simulink model "MdXXHolderChk"  (R2024b)
settings: Solver=FixedStepDiscrete  StartTime=0.0  StopTime=10.0  FixedStep=0.01  RelTol=1e-3
undefined symbols (not defined in the file or in its folder): KeSMSwAcsMd32SecRwLtStBkReclnUpwdDnwdPos1_Val, KeSMSwAcsMd53SecRwRtStBkReclnUpwdDnwdPos1_Val, SeatChldLkSt
libraries: simulink x41
(part 2 of 5)

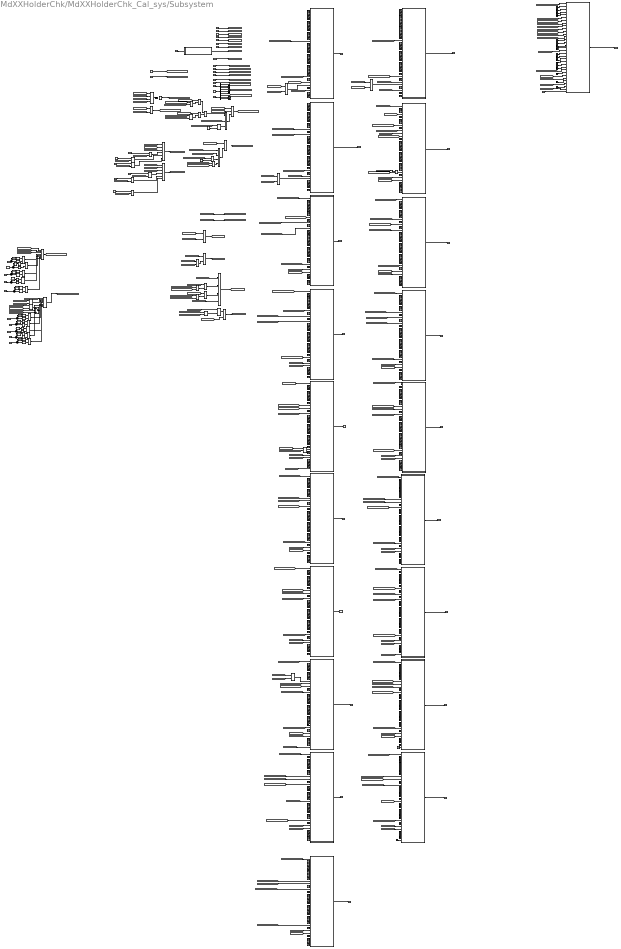
== system MdXXHolderChk/MdXXHolderChk_Cal_sys/Subsystem ==
  note: 零重力模式，二排任意一个电机没到位，模式直接停止
  ChldLkRspFlgL_Val_read : Inport
  ChldLkRspFlgR_Val_read : Inport  Port=2
  PassSeatOccupied_Val_read : Inport  Port=3
  R3LMdSeatOccupied_Val_read : Inport  Port=4
  R3RMdSeatOccupied_Val_read : Inport  Port=5
  R2LMdSeatOccupied_Val_read : Inport  Port=6
  R2RMdSeatOccupied_Val_read : Inport  Port=7
  StNumFlg_Is7s_read : Inport  Port=8
  IfVeSMSbThdRwLtStCshnFldUpwdDnwdMovConfig_Val_read : Inport  Port=9
  IfVeSMSuThdRwLtStCshnFldUpwdDnwdPos_Val_read : Inport  Port=10
  IfVeSMSuThdRwRtStCshnFldUpwdDnwdPos_Val_read : Inport  Port=11
  IfVeSMSbThdRwRtStCshnFldUpwdDnwdMovConfig_Val_read : Inport  Port=12
  IfVeSMSuSecRwLtStBkReclnUpwdDnwdPos_Val_read : Inport  Port=13
  IfVeSMSuSecRwRtStBkReclnUpwdDnwdPos_Val_read : Inport  Port=14
  Md8R2LBkReclnUpwdDnwdTrgtPosCalib_TrgtPosArray_read : Inport  Port=15
  Md8R2RBkReclnUpwdDnwdTrgtPosCalib_TrgtPosArray_read : Inport  Port=16
  Md9R2RBkReclnUpwdDnwdTrgtPosCalib_TrgtPosArray_read : Inport  Port=17
  ThdRwLtStChldLkReq_Val_read : Inport  Port=18
  KeSMSwAcsMd32SecRwLtStBkReclnUpwdDnwdPos1 : Inport  Port=19
  KeSMSwAcsMd53SecRwRtStBkReclnUpwdDnwdPos1 : Inport  Port=20
  Md61PassStTrgtIsFld_Val_read : Inport  Port=21
  Md61ThdRwLtStTrgtIsFld_Val_read : Inport  Port=22
  Md61ThdRwRtStTrgtIsFld_Val_read : Inport  Port=23
  Md62PassStTrgtIsFld_Val_read : Inport  Port=24
  Md62ThdRwLtStTrgtIsFld_Val_read : Inport  Port=25
  Md62ThdRwRtStTrgtIsFld_Val_read : Inport  Port=26
  BkReclinctrlquitflagL_Val_read : Inport  Port=27
  BkReclnquitflag_Val_read : Inport  Port=28
  FwdBkwdquitflag_Val_read : Inport  Port=29
  FwdBkwdquitflagL_Val_read : Inport  Port=30
  LgrstDwwdUpwdquitflagL_Val_read : Inport  Port=31
  LgrstInwdOtwdquitflagL_Val_read : Inport  Port=32
  LgrstInwrdOutwdquitflag_Val_read : Inport  Port=33
  LgrstUpwdDnwdquitflag_Val_read : Inport  Port=34
  Zeroquitflag_Val_read : Inport  Port=35
  zeroquitflagL_Val_read : Inport  Port=36
  modestate32_Val_read : Inport  Port=37
  Compare To Constant{,2,4,6,8,10,12,14,16,18} (10 alike) : simulink/Logic and Bit Operations/Compare To Constant  relop===  const=0  OutDataTypeStr=boolean
  Compare To Constant{1,3,5,7,9,11,13,15,17,19} (10 alike) : simulink/Logic and Bit Operations/Compare To Constant  relop===  const=1  OutDataTypeStr=boolean
  Constant : Constant  Value=0  OutDataTypeStr=boolean
  Constant1 : Constant  Value=40  OutDataTypeStr=uint16
  Constant3 : Constant  Value=40  OutDataTypeStr=uint16
  Demux : Demux  Outputs=3
  Demux1 : Demux  Outputs=3
  Demux2 : Demux  Outputs=3
  Ground{,1..3,8..11,13..18,20..21,23} (17 alike) : Ground
  Ground_{1..26,28..41,43,45..56,58,61..64,66..72,75,77..88,90,93..96,98..104,107,109..113,115..120,122,125..127,130..135,139,141..152,154,157..159,162..168,171,173..184,186,189..192,194..200,203,205..216,218,221..224,226..231,233,235,237..248,250,253..256,258..263,265,267,269..280,282,285..288,291,293..295,297,301..312,314,317..331,333..344,346,349,351..352,354..359,361,363,365..376,378,381..384,386..391,393,395,397..408,410,413..416,418..424,427,429..440,442,445..447,450..456,459,461..472,474,477..480,482..488,491,493..504,506,509..512,514..519,523,525..535,538,541..543,546..552,555,557..561,563..568,570,573..576,578..583,585,587,589..600,602,605..607} (472 alike) : Ground
  Logical Operator{,1,5,8,10..11,13,16..17,46,79,82,86} (13 alike) : Logic  Operator=OR  AllPortsSameDT=off  OutDataTypeStr=boolean
  Logical Operator{6..7,12,14..15,18,20..34,45,83} (23 alike) : Logic  AllPortsSameDT=off  OutDataTypeStr=boolean
  Logical Operator19 : Logic  Operator=OR  Inputs=6  AllPortsSameDT=off  OutDataTypeStr=boolean
  Logical Operator2 : Logic  Operator=OR  Inputs=8  AllPortsSameDT=off  OutDataTypeStr=boolean
  Logical Operator3 : Logic  Operator=OR  Inputs=4  AllPortsSameDT=off  OutDataTypeStr=boolean
  Logical Operator4 : Logic  Operator=OR  Inputs=6  AllPortsSameDT=off  OutDataTypeStr=boolean
  Logical Operator78 : Logic  Inputs=4  AllPortsSameDT=off  OutDataTypeStr=boolean
  Logical Operator81 : Logic  Operator=OR  Inputs=8  AllPortsSameDT=off  OutDataTypeStr=boolean
  Logical Operator84 : Logic  Operator=OR  Inputs=3  AllPortsSameDT=off  OutDataTypeStr=boolean
  Logical Operator85 : Logic  Inputs=3  AllPortsSameDT=off  OutDataTypeStr=boolean
  Logical Operator9 : Logic  Operator=OR  Inputs=4  AllPortsSameDT=off  OutDataTypeStr=boolean
  Relational Operator{1..8} (8 alike) : RelationalOperator  Operator=>  OutDataTypeStr=boolean  RndMeth=Simplest  InputSameDT=off
  Subsystem : Subsystem
  Subsystem1 : Subsystem
  Subsystem10 : Subsystem
  Subsystem11 : Subsystem
  Subsystem12 : Subsystem
  Subsystem13 : Subsystem
  Subsystem14 : Subsystem
  Subsystem15 : Subsystem
  Subsystem16 : Subsystem
  Subsystem17 : Subsystem
  Subsystem18 : Subsystem
  Subsystem19 : Subsystem
  Subsystem2 : Subsystem
  Subsystem20 : Subsystem
  Subsystem3 : Subsystem
  Subsystem4 : Subsystem
  Subsystem5 : Subsystem
  Subsystem6 : Subsystem
  Subsystem7 : Subsystem
  Subsystem8 : Subsystem
  Subsystem9 : Subsystem
  Switch19 : Switch  Criteria=u2 > Threshold  SaturateOnIntegerOverflow=off  InputSameDT=off
  Terminator{,1..6} (7 alike) : Terminator
  Unit Delay{,1..9} (10 alike) : UnitDelay  SampleTime=-1  HasFrameUpgradeWarning=on
  MdXXPassStBkReclnHolderInfo_Val_write : Outport  VectorParamsAs1DForOutWhenUnconnected=off
      settings: EnsureOutportIsVirtual=on
  MdXXPassStCshnFldHolderInfo_Val_write : Outport  Port=2  VectorParamsAs1DForOutWhenUnconnected=off
      settings: EnsureOutportIsVirtual=on
  MdXXPassStFwdBkwdHolderInfo_Val_write : Outport  Port=3  VectorParamsAs1DForOutWhenUnconnected=off
      settings: EnsureOutportIsVirtual=on
  MdXXSecRwLtStBkReclnHolderInfo_Val_write : Outport  Port=4  VectorParamsAs1DForOutWhenUnconnected=off
      settings: EnsureOutportIsVirtual=on
  MdXXSecRwLtStFwdBkwdHolderInfo_Val_write : Outport  Port=5  VectorParamsAs1DForOutWhenUnconnected=off
      settings: EnsureOutportIsVirtual=on
  MdXXSecRwLtStLgrstInwdOtwdHolderInfo_Val_write : Outport  Port=6  VectorParamsAs1DForOutWhenUnconnected=off
      settings: EnsureOutportIsVirtual=on
  MdXXSecRwLtStLgrstUpwdDnwdHolderInfo_Val_write : Outport  Port=7  VectorParamsAs1DForOutWhenUnconnected=off
      settings: EnsureOutportIsVirtual=on
  MdXXSecRwLtStZeroHolderInfo_Val_write : Outport  Port=8  VectorParamsAs1DForOutWhenUnconnected=off
      settings: EnsureOutportIsVirtual=on
  MdXXSecRwRtStBkReclnEnHolderInfo_Val_write : Outport  Port=9  VectorParamsAs1DForOutWhenUnconnected=off
      settings: EnsureOutportIsVirtual=on
  MdXXSecRwRtStFwdBkwdHolderInfo_Val_write : Outport  Port=10  VectorParamsAs1DForOutWhenUnconnected=off
      settings: EnsureOutportIsVirtual=on
  MdXXSecRwRtStLgrstInwdOtwdHolderInfo_Val_write : Outport  Port=11  VectorParamsAs1DForOutWhenUnconnected=off
      settings: EnsureOutportIsVirtual=on
  MdXXSecRwRtStLgrstUpwdDnwdHolderInfo_Val_write : Outport  Port=12  VectorParamsAs1DForOutWhenUnconnected=off
      settings: EnsureOutportIsVirtual=on
  MdXXSecRwRtStZeroHolderInfo_Val_write : Outport  Port=13  VectorParamsAs1DForOutWhenUnconnected=off
      settings: EnsureOutportIsVirtual=on
  MdXXThdRwLtStBkReclnHolderInfo_Val_write : Outport  Port=14  VectorParamsAs1DForOutWhenUnconnected=off
      settings: EnsureOutportIsVirtual=on
  MdXXThdRwLtStCshnFldHolderInfo_Val_write : Outport  Port=15  VectorParamsAs1DForOutWhenUnconnected=off
      settings: EnsureOutportIsVirtual=on
  MdXXThdRwLtStFwdBkwdHolderInfo_Val_write : Outport  Port=16  VectorParamsAs1DForOutWhenUnconnected=off
      settings: EnsureOutportIsVirtual=on
  MdXXThdRwRtStBkReclnHolderInfo_Val_write : Outport  Port=17  VectorParamsAs1DForOutWhenUnconnected=off
      settings: EnsureOutportIsVirtual=on
  MdXXThdRwRtStCshnFldHolderInfo_Val_write : Outport  Port=18  VectorParamsAs1DForOutWhenUnconnected=off
      settings: EnsureOutportIsVirtual=on
  MdXXThdRwRtStFwdBkwdHolderInfo_Val_write : Outport  Port=19  VectorParamsAs1DForOutWhenUnconnected=off
      settings: EnsureOutportIsVirtual=on
  MdXXHolderInfo_Val_write : Outport  Port=20  VectorParamsAs1DForOutWhenUnconnected=off
      settings: EnsureOutportIsVirtual=on
  wires:
  Subsystem/1(MdXXHolder) -> MdXXPassStBkReclnHolderInfo_Val_write/1
  Subsystem18/1(MdXXHolder) -> MdXXPassStCshnFldHolderInfo_Val_write/1
  Subsystem1/1(MdXXHolder) -> MdXXPassStFwdBkwdHolderInfo_Val_write/1
  Subsystem17/1(MdXXHolder) -> MdXXSecRwLtStBkReclnHolderInfo_Val_write/1
  Subsystem2/1(MdXXHolder) -> MdXXSecRwLtStFwdBkwdHolderInfo_Val_write/1
  Subsystem16/1(MdXXHolder) -> MdXXSecRwLtStLgrstInwdOtwdHolderInfo_Val_write/1
  Subsystem3/1(MdXXHolder) -> MdXXSecRwLtStLgrstUpwdDnwdHolderInfo_Val_write/1
  Subsystem15/1(MdXXHolder) -> MdXXSecRwLtStZeroHolderInfo_Val_write/1
  Subsystem4/1(MdXXHolder) -> MdXXSecRwRtStBkReclnEnHolderInfo_Val_write/1
  Subsystem14/1(MdXXHolder) -> MdXXSecRwRtStFwdBkwdHolderInfo_Val_write/1
  Subsystem5/1(MdXXHolder) -> MdXXSecRwRtStLgrstInwdOtwdHolderInfo_Val_write/1
  Subsystem13/1(MdXXHolder) -> MdXXSecRwRtStLgrstUpwdDnwdHolderInfo_Val_write/1
  Subsystem6/1(MdXXHolder) -> MdXXSecRwRtStZeroHolderInfo_Val_write/1
  Subsystem9/1(MdXXHolder) -> MdXXThdRwLtStBkReclnHolderInfo_Val_write/1
  Subsystem7/1(MdXXHolder) -> MdXXThdRwLtStCshnFldHolderInfo_Val_write/1
  Subsystem12/1(MdXXHolder) -> MdXXThdRwLtStFwdBkwdHolderInfo_Val_write/1
  Subsystem8/1(MdXXHolder) -> MdXXThdRwRtStBkReclnHolderInfo_Val_write/1
  Subsystem11/1(MdXXHolder) -> MdXXThdRwRtStCshnFldHolderInfo_Val_write/1
  Subsystem10/1(MdXXHolder) -> MdXXThdRwRtStFwdBkwdHolderInfo_Val_write/1
  ChldLkRspFlgL_Val_read/1 -> [ChldLkRspFlgL]
  ChldLkRspFlgR_Val_read/1 -> [ChldLkRspFlgR]
  PassSeatOccupied_Val_read/1 -> [PassSeatOccupied]
  R3LMdSeatOccupied_Val_read/1 -> [R3LMdSeatOccupied]
  R3RMdSeatOccupied_Val_read/1 -> [R3RMdSeatOccupied]
  Ground_1/1 -> Subsystem/1(Md1HoldReq)
  Ground_2/1 -> Subsystem/2(Md2HoldReq)
  Ground_3/1 -> Subsystem/3(Md3HoldReq)
  Ground_4/1 -> Subsystem/4(Md4HoldReq)
  Ground_5/1 -> Subsystem/5(Md5HoldReq)
  Ground_6/1 -> Subsystem/6(Md6HoldReq)
  Ground_7/1 -> Subsystem/7(Md7HoldReq)
  Ground_8/1 -> Subsystem/8(Md8HoldReq)
  Ground_9/1 -> Subsystem/9(Md9HoldReq)
  Ground_10/1 -> Subsystem/10(Md10HoldReq)
  Ground_11/1 -> Subsystem/11(Md11HoldReq)
  Ground_13/1 -> Subsystem/13(Md13HoldReq)
  Ground_14/1 -> Subsystem/14(Md14HoldReq)
  Ground_15/1 -> Subsystem/15(Md15HoldReq)
  Ground_16/1 -> Subsystem/16(Md16HoldReq)
  Ground_17/1 -> Subsystem/17(Md17HoldReq)
  Ground_18/1 -> Subsystem/18(Md18HoldReq)
  Ground_19/1 -> Subsystem/19(Md19HoldReq)
  Ground_20/1 -> Subsystem/20(Md20HoldReq)
  Ground_21/1 -> Subsystem/21(Md21HoldReq)
  Ground_22/1 -> Subsystem/22(Md22HoldReq)
  Ground_23/1 -> Subsystem/23(Md23HoldReq)
  Ground_24/1 -> Subsystem/24(Md24HoldReq)
  [Md56Stop] -> Subsystem/25(Md25HoldReq)
  Ground_26/1 -> Subsystem/26(Md26HoldReq)
  Ground_29/1 -> Subsystem/29(Md29HoldReq)
  [PassSeatOccupied] -> Subsystem/30(Md30HoldReq)
  Ground_31/1 -> Subsystem/31(Md31HoldReq)
  Ground_32/1 -> Subsystem/32(Md32HoldReq)
  Ground_33/1 -> Subsystem1/1(Md1HoldReq)
  Ground_34/1 -> Subsystem1/2(Md2HoldReq)
  Ground_35/1 -> Subsystem1/3(Md3HoldReq)
  Ground_36/1 -> Subsystem1/4(Md4HoldReq)
  Ground_37/1 -> Subsystem1/5(Md5HoldReq)
  Ground_38/1 -> Subsystem1/6(Md6HoldReq)
  Ground_39/1 -> Subsystem1/7(Md7HoldReq)
  Ground_40/1 -> Subsystem1/8(Md8HoldReq)
  Ground_41/1 -> Subsystem1/9(Md9HoldReq)
  Ground_43/1 -> Subsystem1/11(Md11HoldReq)
  Ground_45/1 -> Subsystem1/13(Md13HoldReq)
  Ground_46/1 -> Subsystem1/14(Md14HoldReq)
  Ground_47/1 -> Subsystem1/15(Md15HoldReq)
  Ground_48/1 -> Subsystem1/16(Md16HoldReq)
  Ground_49/1 -> Subsystem1/17(Md17HoldReq)
  Ground_50/1 -> Subsystem1/18(Md18HoldReq)
  Ground_51/1 -> Subsystem1/19(Md19HoldReq)
  Ground_52/1 -> Subsystem1/20(Md20HoldReq)
  Ground_53/1 -> Subsystem1/21(Md21HoldReq)
  Ground_54/1 -> Subsystem1/22(Md22HoldReq)
  Ground_55/1 -> Subsystem1/23(Md23HoldReq)
  Ground_56/1 -> Subsystem1/24(Md24HoldReq)
  [Md56Stop] -> Subsystem1/25(Md25HoldReq)
  Ground_58/1 -> Subsystem1/26(Md26HoldReq)
  [Md27Stop] -> Subsystem1/27(Md27HoldReq)
  Ground_61/1 -> Subsystem1/29(Md29HoldReq)
  Ground_62/1 -> Subsystem1/30(Md30HoldReq)
  Ground_63/1 -> Subsystem1/31(Md31HoldReq)
  Ground_64/1 -> Subsystem1/32(Md32HoldReq)
  [Md1Stop] -> Subsystem10/1(Md1HoldReq)
  Ground_66/1 -> Subsystem10/2(Md2HoldReq)
  Ground_67/1 -> Subsystem10/3(Md3HoldReq)
  Ground_68/1 -> Subsystem10/4(Md4HoldReq)
  Ground_69/1 -> Subsystem10/5(Md5HoldReq)
  Ground_70/1 -> Subsystem10/6(Md6HoldReq)
  Ground_71/1 -> Subsystem10/7(Md7HoldReq)
  Ground_72/1 -> Subsystem10/8(Md8HoldReq)
  [Md10Stop] -> Subsystem10/10(Md10HoldReq)
  Ground_75/1 -> Subsystem10/11(Md11HoldReq)
  Ground_77/1 -> Subsystem10/13(Md13HoldReq)
  Ground_78/1 -> Subsystem10/14(Md14HoldReq)
  Ground_79/1 -> Subsystem10/15(Md15HoldReq)
  Ground_80/1 -> Subsystem10/16(Md16HoldReq)
  Ground_81/1 -> Subsystem10/17(Md17HoldReq)
  Ground_82/1 -> Subsystem10/18(Md18HoldReq)
  Ground_83/1 -> Subsystem10/19(Md19HoldReq)
  Ground_84/1 -> Subsystem10/20(Md20HoldReq)
  Ground_85/1 -> Subsystem10/21(Md21HoldReq)
  Ground_86/1 -> Subsystem10/22(Md22HoldReq)
  Ground_87/1 -> Subsystem10/23(Md23HoldReq)
  Ground_88/1 -> Subsystem10/24(Md24HoldReq)
  [Md56Stop] -> Subsystem10/25(Md25HoldReq)
  Ground_90/1 -> Subsystem10/26(Md26HoldReq)
  Ground_93/1 -> Subsystem10/29(Md29HoldReq)
  Ground_94/1 -> Subsystem10/30(Md30HoldReq)
  Ground_95/1 -> Subsystem10/31(Md31HoldReq)
  Ground_96/1 -> Subsystem10/32(Md32HoldReq)
  [Md1Stop] -> Subsystem11/1(Md1HoldReq)
  Ground_98/1 -> Subsystem11/2(Md2HoldReq)
  Ground_99/1 -> Subsystem11/3(Md3HoldReq)
  Ground_100/1 -> Subsystem11/4(Md4HoldReq)
  Ground_101/1 -> Subsystem11/5(Md5HoldReq)
  Ground_102/1 -> Subsystem11/6(Md6HoldReq)
  Ground_103/1 -> Subsystem11/7(Md7HoldReq)
  Ground_104/1 -> Subsystem11/8(Md8HoldReq)
  [Md10Stop] -> Subsystem11/10(Md10HoldReq)
  Ground_107/1 -> Subsystem11/11(Md11HoldReq)
  Ground_109/1 -> Subsystem11/13(Md13HoldReq)
  Ground_110/1 -> Subsystem11/14(Md14HoldReq)
  Ground_111/1 -> Subsystem11/15(Md15HoldReq)
  Ground_112/1 -> Subsystem11/16(Md16HoldReq)
  Ground_113/1 -> Subsystem11/17(Md17HoldReq)
  [R3RMdSeatOccupied] -> Subsystem11/18(Md18HoldReq)
  Ground_115/1 -> Subsystem11/19(Md19HoldReq)
  Ground_116/1 -> Subsystem11/20(Md20HoldReq)
  Ground_117/1 -> Subsystem11/21(Md21HoldReq)
  Ground_118/1 -> Subsystem11/22(Md22HoldReq)
  Ground_119/1 -> Subsystem11/23(Md23HoldReq)
  Ground_120/1 -> Subsystem11/24(Md24HoldReq)
  [Md56Stop] -> Subsystem11/25(Md25HoldReq)
  Ground_122/1 -> Subsystem11/26(Md26HoldReq)
  Ground_125/1 -> Subsystem11/29(Md29HoldReq)
  Ground_126/1 -> Subsystem11/30(Md30HoldReq)
  Ground_127/1 -> Subsystem11/31(Md31HoldReq)
  [Md1Stop] -> Subsystem12/1(Md1HoldReq)
  Ground_130/1 -> Subsystem12/2(Md2HoldReq)
  Ground_131/1 -> Subsystem12/3(Md3HoldReq)
  Ground_132/1 -> Subsystem12/4(Md4HoldReq)
  Ground_133/1 -> Subsystem12/5(Md5HoldReq)
  Ground_134/1 -> Subsystem12/6(Md6HoldReq)
  Ground_135/1 -> Subsystem12/7(Md7HoldReq)
  [Md9Stop] -> Subsystem12/9(Md9HoldReq)
  [Md10Stop] -> Subsystem12/10(Md10HoldReq)
  Ground_139/1 -> Subsystem12/11(Md11HoldReq)
  Ground_141/1 -> Subsystem12/13(Md13HoldReq)
  Ground_142/1 -> Subsystem12/14(Md14HoldReq)
  Ground_143/1 -> Subsystem12/15(Md15HoldReq)
  Ground_144/1 -> Subsystem12/16(Md16HoldReq)
  Ground_145/1 -> Subsystem12/17(Md17HoldReq)
  Ground_146/1 -> Subsystem12/18(Md18HoldReq)
  Ground_147/1 -> Subsystem12/19(Md19HoldReq)
  Ground_148/1 -> Subsystem12/20(Md20HoldReq)
  Ground_149/1 -> Subsystem12/21(Md21HoldReq)
  Ground_150/1 -> Subsystem12/22(Md22HoldReq)
  Ground_151/1 -> Subsystem12/23(Md23HoldReq)
  Ground_152/1 -> Subsystem12/24(Md24HoldReq)
  [Md56Stop] -> Subsystem12/25(Md25HoldReq)
  Ground_154/1 -> Subsystem12/26(Md26HoldReq)
  Ground_157/1 -> Subsystem12/29(Md29HoldReq)
  Ground_158/1 -> Subsystem12/30(Md30HoldReq)
  Ground_159/1 -> Subsystem12/31(Md31HoldReq)
  Ground_28/1 -> Subsystem12/32(Md32HoldReq)
  [Md1Stop] -> Subsystem13/1(Md1HoldReq)
  Ground_162/1 -> Subsystem13/2(Md2HoldReq)
  Ground_163/1 -> Subsystem13/3(Md3HoldReq)
  Ground_164/1 -> Subsystem13/4(Md4HoldReq)
  Ground_165/1 -> Subsystem13/5(Md5HoldReq)
  Ground_166/1 -> Subsystem13/6(Md6HoldReq)
  Ground_167/1 -> Subsystem13/7(Md7HoldReq)
  Ground_168/1 -> Subsystem13/8(Md8HoldReq)
  [Md9Stop] -> Subsystem13/9(Md9HoldReq)
  [Md10Stop] -> Subsystem13/10(Md10HoldReq)
  Ground_171/1 -> Subsystem13/11(Md11HoldReq)
  Ground_173/1 -> Subsystem13/13(Md13HoldReq)
  Ground_174/1 -> Subsystem13/14(Md14HoldReq)
  Ground_175/1 -> Subsystem13/15(Md15HoldReq)
  Ground_176/1 -> Subsystem13/16(Md16HoldReq)
  Ground_177/1 -> Subsystem13/17(Md17HoldReq)
  Ground_178/1 -> Subsystem13/18(Md18HoldReq)
  Ground_179/1 -> Subsystem13/19(Md19HoldReq)
  Ground_180/1 -> Subsystem13/20(Md20HoldReq)
  Ground_181/1 -> Subsystem13/21(Md21HoldReq)
  Ground_182/1 -> Subsystem13/22(Md22HoldReq)
  Ground_183/1 -> Subsystem13/23(Md23HoldReq)
  Ground_184/1 -> Subsystem13/24(Md24HoldReq)
  [Md56Stop] -> Subsystem13/25(Md25HoldReq)
  Ground_186/1 -> Subsystem13/26(Md26HoldReq)
  Ground_189/1 -> Subsystem13/29(Md29HoldReq)
  Ground_190/1 -> Subsystem13/30(Md30HoldReq)
  Ground_191/1 -> Subsystem13/31(Md31HoldReq)
  Ground_192/1 -> Subsystem13/32(Md32HoldReq)
  [Md1Stop] -> Subsystem14/1(Md1HoldReq)
  Ground_194/1 -> Subsystem14/2(Md2HoldReq)
  Ground_195/1 -> Subsystem14/3(Md3HoldReq)
  Ground_196/1 -> Subsystem14/4(Md4HoldReq)
  Ground_197/1 -> Subsystem14/5(Md5HoldReq)
  Ground_198/1 -> Subsystem14/6(Md6HoldReq)
  Ground_199/1 -> Subsystem14/7(Md7HoldReq)
  Ground_200/1 -> Subsystem14/8(Md8HoldReq)
  [Md9Stop] -> Subsystem14/9(Md9HoldReq)
  [Md10Stop] -> Subsystem14/10(Md10HoldReq)
  Ground_203/1 -> Subsystem14/11(Md11HoldReq)
  Ground_205/1 -> Subsystem14/13(Md13HoldReq)
  Ground_206/1 -> Subsystem14/14(Md14HoldReq)
  Ground_207/1 -> Subsystem14/15(Md15HoldReq)
  Ground_208/1 -> Subsystem14/16(Md16HoldReq)
  Ground_209/1 -> Subsystem14/17(Md17HoldReq)
  Ground_210/1 -> Subsystem14/18(Md18HoldReq)
  Ground_211/1 -> Subsystem14/19(Md19HoldReq)
  Ground_212/1 -> Subsystem14/20(Md20HoldReq)
  Ground_213/1 -> Subsystem14/21(Md21HoldReq)
  Ground_214/1 -> Subsystem14/22(Md22HoldReq)
  Ground_215/1 -> Subsystem14/23(Md23HoldReq)
  Ground_216/1 -> Subsystem14/24(Md24HoldReq)
  [Md56Stop] -> Subsystem14/25(Md25HoldReq)
  Ground_218/1 -> Subsystem14/26(Md26HoldReq)
  Ground_221/1 -> Subsystem14/29(Md29HoldReq)
  Ground_222/1 -> Subsystem14/30(Md30HoldReq)
  Ground_223/1 -> Subsystem14/31(Md31HoldReq)
  Ground_224/1 -> Subsystem14/32(Md32HoldReq)
  [Md1Stop] -> Subsystem15/1(Md1HoldReq)
  Ground_226/1 -> Subsystem15/2(Md2HoldReq)
  Ground_227/1 -> Subsystem15/3(Md3HoldReq)
  Ground_228/1 -> Subsystem15/4(Md4HoldReq)
  Ground_229/1 -> Subsystem15/5(Md5HoldReq)
  Ground_230/1 -> Subsystem15/6(Md6HoldReq)
  Ground_231/1 -> Subsystem15/7(Md7HoldReq)
  [Md8Stop] -> Subsystem15/8(Md8HoldReq)
  Ground_233/1 -> Subsystem15/9(Md9HoldReq)
  Ground_235/1 -> Subsystem15/11(Md11HoldReq)
  Ground_237/1 -> Subsystem15/13(Md13HoldReq)
  Ground_238/1 -> Subsystem15/14(Md14HoldReq)
  Ground_239/1 -> Subsystem15/15(Md15HoldReq)
  Ground_240/1 -> Subsystem15/16(Md16HoldReq)
  Ground_241/1 -> Subsystem15/17(Md17HoldReq)
  Ground_242/1 -> Subsystem15/18(Md18HoldReq)
  Ground_243/1 -> Subsystem15/19(Md19HoldReq)
  Ground_244/1 -> Subsystem15/20(Md20HoldReq)
  Ground_245/1 -> Subsystem15/21(Md21HoldReq)
  Ground_246/1 -> Subsystem15/22(Md22HoldReq)
  Ground_247/1 -> Subsystem15/23(Md23HoldReq)
  Ground_248/1 -> Subsystem15/24(Md24HoldReq)
  [Md56Stop] -> Subsystem15/25(Md25HoldReq)
  Ground_250/1 -> Subsystem15/26(Md26HoldReq)
  Ground_253/1 -> Subsystem15/29(Md29HoldReq)
  Ground_254/1 -> Subsystem15/30(Md30HoldReq)
  Ground_255/1 -> Subsystem15/31(Md31HoldReq)
  Ground_256/1 -> Subsystem15/32(Md32HoldReq)
  [Md1Stop] -> Subsystem16/1(Md1HoldReq)
  Ground_258/1 -> Subsystem16/2(Md2HoldReq)
  Ground_259/1 -> Subsystem16/3(Md3HoldReq)
  Ground_260/1 -> Subsystem16/4(Md4HoldReq)
  Ground_261/1 -> Subsystem16/5(Md5HoldReq)
  Ground_262/1 -> Subsystem16/6(Md6HoldReq)
  Ground_263/1 -> Subsystem16/7(Md7HoldReq)
  Ground_265/1 -> Subsystem16/9(Md9HoldReq)
  [Md10Stop] -> Subsystem16/10(Md10HoldReq)
  Ground_267/1 -> Subsystem16/11(Md11HoldReq)
  Ground_269/1 -> Subsystem16/13(Md13HoldReq)
  Ground_270/1 -> Subsystem16/14(Md14HoldReq)
  Ground_271/1 -> Subsystem16/15(Md15HoldReq)
  Ground_272/1 -> Subsystem16/16(Md16HoldReq)
  Ground_273/1 -> Subsystem16/17(Md17HoldReq)
  Ground_274/1 -> Subsystem16/18(Md18HoldReq)
  Ground_275/1 -> Subsystem16/19(Md19HoldReq)
  Ground_276/1 -> Subsystem16/20(Md20HoldReq)
  Ground_277/1 -> Subsystem16/21(Md21HoldReq)
  Ground_278/1 -> Subsystem16/22(Md22HoldReq)
  Ground_279/1 -> Subsystem16/23(Md23HoldReq)
  Ground_280/1 -> Subsystem16/24(Md24HoldReq)
  [Md56Stop] -> Subsystem16/25(Md25HoldReq)
  Ground_282/1 -> Subsystem16/26(Md26HoldReq)
  [Md27Stop] -> Subsystem16/27(Md27HoldReq)
  Ground_285/1 -> Subsystem16/29(Md29HoldReq)
  Ground_286/1 -> Subsystem16/30(Md30HoldReq)
  Ground_287/1 -> Subsystem16/31(Md31HoldReq)
  Ground_288/1 -> Subsystem16/32(Md32HoldReq)
  Ground_291/1 -> Subsystem17/3(Md3HoldReq)
  [ChldLkRspFlgL] -> Subsystem17/4(Md4HoldReq)
  Ground_293/1 -> Subsystem17/5(Md5HoldReq)
  Ground_294/1 -> Subsystem17/6(Md6HoldReq)
  Ground_295/1 -> Subsystem17/7(Md7HoldReq)
  Ground_297/1 -> Subsystem17/9(Md9HoldReq)
  [ChldLkRspFlgL] -> Subsystem17/11(Md11HoldReq)
  Ground_301/1 -> Subsystem17/13(Md13HoldReq)
  Ground_302/1 -> Subsystem17/14(Md14HoldReq)
  Ground_303/1 -> Subsystem17/15(Md15HoldReq)
  Ground_304/1 -> Subsystem17/16(Md16HoldReq)
  Ground_305/1 -> Subsystem17/17(Md17HoldReq)
  Ground_306/1 -> Subsystem17/18(Md18HoldReq)
  Ground_307/1 -> Subsystem17/19(Md19HoldReq)
  Ground_308/1 -> Subsystem17/20(Md20HoldReq)
  Ground_309/1 -> Subsystem17/21(Md21HoldReq)
  Ground_310/1 -> Subsystem17/22(Md22HoldReq)
  Ground_311/1 -> Subsystem17/23(Md23HoldReq)
  Ground_312/1 -> Subsystem17/24(Md24HoldReq)
  Ground_314/1 -> Subsystem17/26(Md26HoldReq)
  [Md27Stop] -> Subsystem17/27(Md27HoldReq)
  Ground_317/1 -> Subsystem17/29(Md29HoldReq)
  Ground_318/1 -> Subsystem17/30(Md30HoldReq)
  Ground_319/1 -> Subsystem17/31(Md31HoldReq)
  Ground_320/1 -> Subsystem17/32(Md32HoldReq)
  Ground_321/1 -> Subsystem18/1(Md1HoldReq)
  Ground_322/1 -> Subsystem18/2(Md2HoldReq)
  Ground_323/1 -> Subsystem18/3(Md3HoldReq)
  Ground_324/1 -> Subsystem18/4(Md4HoldReq)
  Ground_325/1 -> Subsystem18/5(Md5HoldReq)
  Ground_326/1 -> Subsystem18/6(Md6HoldReq)
  Ground_327/1 -> Subsystem18/7(Md7HoldReq)
  Ground_328/1 -> Subsystem18/8(Md8HoldReq)
  Ground_329/1 -> Subsystem18/9(Md9HoldReq)
  Ground_330/1 -> Subsystem18/10(Md10HoldReq)
  Ground_331/1 -> Subsystem18/11(Md11HoldReq)
  [Md12Stop] -> Subsystem18/12(Md12HoldReq)
  Ground_333/1 -> Subsystem18/13(Md13HoldReq)
  Ground_334/1 -> Subsystem18/14(Md14HoldReq)
  Ground_335/1 -> Subsystem18/15(Md15HoldReq)
  Ground_336/1 -> Subsystem18/16(Md16HoldReq)
  Ground_337/1 -> Subsystem18/17(Md17HoldReq)
  Ground_338/1 -> Subsystem18/18(Md18HoldReq)
  Ground_339/1 -> Subsystem18/19(Md19HoldReq)
  Ground_340/1 -> Subsystem18/20(Md20HoldReq)
  Ground_341/1 -> Subsystem18/21(Md21HoldReq)
  Ground_342/1 -> Subsystem18/22(Md22HoldReq)
  Ground_343/1 -> Subsystem18/23(Md23HoldReq)
  Ground_344/1 -> Subsystem18/24(Md24HoldReq)
  [Md56Stop] -> Subsystem18/25(Md25HoldReq)
  Ground_346/1 -> Subsystem18/26(Md26HoldReq)
  [Md27Stop] -> Subsystem18/27(Md27HoldReq)
  Ground_349/1 -> Subsystem18/29(Md29HoldReq)
  [PassSeatOccupied] -> Subsystem18/30(Md30HoldReq)
  Ground_351/1 -> Subsystem18/31(Md31HoldReq)
  Ground_352/1 -> Subsystem18/32(Md32HoldReq)
  [Md1Stop] -> Subsystem2/1(Md1HoldReq)
  Ground_354/1 -> Subsystem2/2(Md2HoldReq)
  Ground_355/1 -> Subsystem2/3(Md3HoldReq)
  Ground_356/1 -> Subsystem2/4(Md4HoldReq)
  Ground_357/1 -> Subsystem2/5(Md5HoldReq)
  Ground_358/1 -> Subsystem2/6(Md6HoldReq)
  Ground_359/1 -> Subsystem2/7(Md7HoldReq)
  Ground_361/1 -> Subsystem2/9(Md9HoldReq)
  Ground_363/1 -> Subsystem2/11(Md11HoldReq)
  [Md12Stop] -> Subsystem2/12(Md12HoldReq)
  Ground_365/1 -> Subsystem2/13(Md13HoldReq)
  Ground_366/1 -> Subsystem2/14(Md14HoldReq)
  Ground_367/1 -> Subsystem2/15(Md15HoldReq)
  Ground_368/1 -> Subsystem2/16(Md16HoldReq)
  Ground_369/1 -> Subsystem2/17(Md17HoldReq)
  Ground_370/1 -> Subsystem2/18(Md18HoldReq)
  Ground_371/1 -> Subsystem2/19(Md19HoldReq)
  Ground_372/1 -> Subsystem2/20(Md20HoldReq)
  Ground_373/1 -> Subsystem2/21(Md21HoldReq)
  Ground_374/1 -> Subsystem2/22(Md22HoldReq)
  Ground_375/1 -> Subsystem2/23(Md23HoldReq)
  Ground_376/1 -> Subsystem2/24(Md24HoldReq)
  [Md56Stop] -> Subsystem2/25(Md25HoldReq)
  Ground_378/1 -> Subsystem2/26(Md26HoldReq)
  Ground_381/1 -> Subsystem2/29(Md29HoldReq)
  Ground_382/1 -> Subsystem2/30(Md30HoldReq)
  Ground_383/1 -> Subsystem2/31(Md31HoldReq)
  Ground_384/1 -> Subsystem2/32(Md32HoldReq)
  [Md1Stop] -> Subsystem3/1(Md1HoldReq)
  Ground_386/1 -> Subsystem3/2(Md2HoldReq)
  Ground_387/1 -> Subsystem3/3(Md3HoldReq)
  Ground_388/1 -> Subsystem3/4(Md4HoldReq)
  Ground_389/1 -> Subsystem3/5(Md5HoldReq)
  Ground_390/1 -> Subsystem3/6(Md6HoldReq)
  Ground_391/1 -> Subsystem3/7(Md7HoldReq)
  Ground_393/1 -> Subsystem3/9(Md9HoldReq)
  [Md10Stop] -> Subsystem3/10(Md10HoldReq)
  Ground_395/1 -> Subsystem3/11(Md11HoldReq)
  Ground_397/1 -> Subsystem3/13(Md13HoldReq)
  Ground_398/1 -> Subsystem3/14(Md14HoldReq)
  Ground_399/1 -> Subsystem3/15(Md15HoldReq)
  Ground_400/1 -> Subsystem3/16(Md16HoldReq)
  Ground_401/1 -> Subsystem3/17(Md17HoldReq)
  Ground_402/1 -> Subsystem3/18(Md18HoldReq)
  Ground_403/1 -> Subsystem3/19(Md19HoldReq)
  Ground_404/1 -> Subsystem3/20(Md20HoldReq)
  Ground_405/1 -> Subsystem3/21(Md21HoldReq)
  Ground_406/1 -> Subsystem3/22(Md22HoldReq)
  Ground_407/1 -> Subsystem3/23(Md23HoldReq)
  Ground_408/1 -> Subsystem3/24(Md24HoldReq)
  [Md56Stop] -> Subsystem3/25(Md25HoldReq)
  Ground_410/1 -> Subsystem3/26(Md26HoldReq)
  Ground_413/1 -> Subsystem3/29(Md29HoldReq)
  Ground_414/1 -> Subsystem3/30(Md30HoldReq)
  Ground_415/1 -> Subsystem3/31(Md31HoldReq)
  Ground_416/1 -> Subsystem3/32(Md32HoldReq)
  Ground_418/1 -> Subsystem4/2(Md2HoldReq)
  Ground_419/1 -> Subsystem4/3(Md3HoldReq)
  Ground_420/1 -> Subsystem4/4(Md4HoldReq)
  Ground_421/1 -> Subsystem4/5(Md5HoldReq)
  Ground_422/1 -> Subsystem4/6(Md6HoldReq)
  Ground_423/1 -> Subsystem4/7(Md7HoldReq)
  Ground_424/1 -> Subsystem4/8(Md8HoldReq)
  [Md10Stop] -> Subsystem4/10(Md10HoldReq)
  Ground_427/1 -> Subsystem4/11(Md11HoldReq)
  Ground_429/1 -> Subsystem4/13(Md13HoldReq)
  Ground_430/1 -> Subsystem4/14(Md14HoldReq)
  Ground_431/1 -> Subsystem4/15(Md15HoldReq)
  Ground_432/1 -> Subsystem4/16(Md16HoldReq)
  Ground_433/1 -> Subsystem4/17(Md17HoldReq)
  Ground_434/1 -> Subsystem4/18(Md18HoldReq)
  Ground_435/1 -> Subsystem4/19(Md19HoldReq)
  Ground_436/1 -> Subsystem4/20(Md20HoldReq)
  Ground_437/1 -> Subsystem4/21(Md21HoldReq)
  Ground_438/1 -> Subsystem4/22(Md22HoldReq)
  Ground_439/1 -> Subsystem4/23(Md23HoldReq)
  Ground_440/1 -> Subsystem4/24(Md24HoldReq)
  Ground_442/1 -> Subsystem4/26(Md26HoldReq)
  Ground_445/1 -> Subsystem4/29(Md29HoldReq)
  Ground_446/1 -> Subsystem4/30(Md30HoldReq)
  Ground_447/1 -> Subsystem4/31(Md31HoldReq)
  [R3RMdSeatOccupied] -> Subsystem4/32(Md32HoldReq)
  [Md1Stop] -> Subsystem5/1(Md1HoldReq)
  Ground_450/1 -> Subsystem5/2(Md2HoldReq)
  Ground_451/1 -> Subsystem5/3(Md3HoldReq)
  Ground_452/1 -> Subsystem5/4(Md4HoldReq)
  Ground_453/1 -> Subsystem5/5(Md5HoldReq)
  Ground_454/1 -> Subsystem5/6(Md6HoldReq)
  Ground_455/1 -> Subsystem5/7(Md7HoldReq)
  Ground_456/1 -> Subsystem5/8(Md8HoldReq)
  [Md9Stop] -> Subsystem5/9(Md9HoldReq)
  Ground_459/1 -> Subsystem5/11(Md11HoldReq)
  Ground_461/1 -> Subsystem5/13(Md13HoldReq)
  Ground_462/1 -> Subsystem5/14(Md14HoldReq)
  Ground_463/1 -> Subsystem5/15(Md15HoldReq)
  Ground_464/1 -> Subsystem5/16(Md16HoldReq)
  Ground_465/1 -> Subsystem5/17(Md17HoldReq)
  Ground_466/1 -> Subsystem5/18(Md18HoldReq)
  Ground_467/1 -> Subsystem5/19(Md19HoldReq)
  Ground_468/1 -> Subsystem5/20(Md20HoldReq)
  Ground_469/1 -> Subsystem5/21(Md21HoldReq)
  Ground_470/1 -> Subsystem5/22(Md22HoldReq)
  Ground_471/1 -> Subsystem5/23(Md23HoldReq)
  Ground_472/1 -> Subsystem5/24(Md24HoldReq)
  [Md56Stop] -> Subsystem5/25(Md25HoldReq)
  Ground_474/1 -> Subsystem5/26(Md26HoldReq)
  Ground_477/1 -> Subsystem5/29(Md29HoldReq)
  Ground_478/1 -> Subsystem5/30(Md30HoldReq)
  Ground_479/1 -> Subsystem5/31(Md31HoldReq)
  Ground_480/1 -> Subsystem5/32(Md32HoldReq)
  [Md1Stop] -> Subsystem6/1(Md1HoldReq)
  Ground_482/1 -> Subsystem6/2(Md2HoldReq)
  Ground_483/1 -> Subsystem6/3(Md3HoldReq)
  Ground_484/1 -> Subsystem6/4(Md4HoldReq)
  Ground_485/1 -> Subsystem6/5(Md5HoldReq)
  Ground_486/1 -> Subsystem6/6(Md6HoldReq)
  Ground_487/1 -> Subsystem6/7(Md7HoldReq)
  Ground_488/1 -> Subsystem6/8(Md8HoldReq)
  [Md9Stop] -> Subsystem6/9(Md9HoldReq)
  Ground_491/1 -> Subsystem6/11(Md11HoldReq)
  [Md12Stop] -> Subsystem6/12(Md12HoldReq)
  Ground_493/1 -> Subsystem6/13(Md13HoldReq)
  Ground_494/1 -> Subsystem6/14(Md14HoldReq)
  Ground_495/1 -> Subsystem6/15(Md15HoldReq)
  Ground_496/1 -> Subsystem6/16(Md16HoldReq)
  Ground_497/1 -> Subsystem6/17(Md17HoldReq)
  Ground_498/1 -> Subsystem6/18(Md18HoldReq)
  Ground_499/1 -> Subsystem6/19(Md19HoldReq)
  Ground_500/1 -> Subsystem6/20(Md20HoldReq)
  Ground_501/1 -> Subsystem6/21(Md21HoldReq)
  Ground_502/1 -> Subsystem6/22(Md22HoldReq)
  Ground_503/1 -> Subsystem6/23(Md23HoldReq)
  Ground_504/1 -> Subsystem6/24(Md24HoldReq)
  [Md56Stop] -> Subsystem6/25(Md25HoldReq)
  Ground_506/1 -> Subsystem6/26(Md26HoldReq)
  Ground_509/1 -> Subsystem6/29(Md29HoldReq)
  Ground_510/1 -> Subsystem6/30(Md30HoldReq)
  Ground_511/1 -> Subsystem6/31(Md31HoldReq)
  Ground_512/1 -> Subsystem6/32(Md32HoldReq)
  [Md1Stop] -> Subsystem7/1(Md1HoldReq)
  Ground_514/1 -> Subsystem7/2(Md2HoldReq)
  Ground_515/1 -> Subsystem7/3(Md3HoldReq)
  Ground_516/1 -> Subsystem7/4(Md4HoldReq)
  Ground_517/1 -> Subsystem7/5(Md5HoldReq)
  Ground_518/1 -> Subsystem7/6(Md6HoldReq)
  Ground_519/1 -> Subsystem7/7(Md7HoldReq)
  Logical Operator5/1 -> Subsystem7/8(Md8HoldReq)
  [Md9Stop] -> Subsystem7/9(Md9HoldReq)
  [Md10Stop] -> Subsystem7/10(Md10HoldReq)
  Ground_523/1 -> Subsystem7/11(Md11HoldReq)
  Ground_525/1 -> Subsystem7/13(Md13HoldReq)
  Ground_526/1 -> Subsystem7/14(Md14HoldReq)
  Ground_527/1 -> Subsystem7/15(Md15HoldReq)
  Ground_528/1 -> Subsystem7/16(Md16HoldReq)
  Ground_529/1 -> Subsystem7/17(Md17HoldReq)
  Ground_530/1 -> Subsystem7/18(Md18HoldReq)
  Ground_531/1 -> Subsystem7/19(Md19HoldReq)
  Ground_532/1 -> Subsystem7/20(Md20HoldReq)
  Ground_533/1 -> Subsystem7/21(Md21HoldReq)
  Ground_534/1 -> Subsystem7/22(Md22HoldReq)
  Ground_535/1 -> Subsystem7/23(Md23HoldReq)
  Ground_25/1 -> Subsystem7/24(Md24HoldReq)
  [Md56Stop] -> Subsystem7/25(Md25HoldReq)
  Ground_538/1 -> Subsystem7/26(Md26HoldReq)
  Ground_541/1 -> Subsystem7/29(Md29HoldReq)
  Ground_542/1 -> Subsystem7/30(Md30HoldReq)
  Ground_543/1 -> Subsystem7/31(Md31HoldReq)
  [R3LMdSeatOccupied] -> Subsystem7/32(Md32HoldReq)
  [Md1Stop] -> Subsystem8/1(Md1HoldReq)
  Ground_546/1 -> Subsystem8/2(Md2HoldReq)
  Ground_547/1 -> Subsystem8/3(Md3HoldReq)
  Ground_548/1 -> Subsystem8/4(Md4HoldReq)
  Ground_549/1 -> Subsystem8/5(Md5HoldReq)
  Ground_550/1 -> Subsystem8/6(Md6HoldReq)
  Ground_551/1 -> Subsystem8/7(Md7HoldReq)
  Ground_552/1 -> Subsystem8/8(Md8HoldReq)
  [Md9Stop] -> Subsystem8/9(Md9HoldReq)
  [Md10Stop] -> Subsystem8/10(Md10HoldReq)
  Ground_555/1 -> Subsystem8/11(Md11HoldReq)
  Ground_557/1 -> Subsystem8/13(Md13HoldReq)
  Ground_558/1 -> Subsystem8/14(Md14HoldReq)
  Ground_559/1 -> Subsystem8/15(Md15HoldReq)
  Ground_560/1 -> Subsystem8/16(Md16HoldReq)
  Ground_561/1 -> Subsystem8/17(Md17HoldReq)
  [R3RMdSeatOccupied] -> Subsystem8/18(Md18HoldReq)
  Ground_563/1 -> Subsystem8/19(Md19HoldReq)
  Ground_564/1 -> Subsystem8/20(Md20HoldReq)
  Ground_565/1 -> Subsystem8/21(Md21HoldReq)
  Ground_566/1 -> Subsystem8/22(Md22HoldReq)
  Ground_567/1 -> Subsystem8/23(Md23HoldReq)
  Ground_568/1 -> Subsystem8/24(Md24HoldReq)
  [Md56Stop] -> Subsystem8/25(Md25HoldReq)
  Ground_570/1 -> Subsystem8/26(Md26HoldReq)
  Ground_573/1 -> Subsystem8/29(Md29HoldReq)
  Ground_574/1 -> Subsystem8/30(Md30HoldReq)
  Ground_575/1 -> Subsystem8/31(Md31HoldReq)
  Ground_576/1 -> Subsystem8/32(Md32HoldReq)
  [Md1Stop] -> Subsystem9/1(Md1HoldReq)
  Ground_578/1 -> Subsystem9/2(Md2HoldReq)
  Ground_579/1 -> Subsystem9/3(Md3HoldReq)
  Ground_580/1 -> Subsystem9/4(Md4HoldReq)
  Ground_581/1 -> Subsystem9/5(Md5HoldReq)
  Ground_582/1 -> Subsystem9/6(Md6HoldReq)
  Ground_583/1 -> Subsystem9/7(Md7HoldReq)
  Ground_585/1 -> Subsystem9/9(Md9HoldReq)
  [Md10Stop] -> Subsystem9/10(Md10HoldReq)
  Ground_587/1 -> Subsystem9/11(Md11HoldReq)
  Ground_589/1 -> Subsystem9/13(Md13HoldReq)
  Ground_590/1 -> Subsystem9/14(Md14HoldReq)
  Ground_591/1 -> Subsystem9/15(Md15HoldReq)
  Ground_592/1 -> Subsystem9/16(Md16HoldReq)
  Ground_593/1 -> Subsystem9/17(Md17HoldReq)
  Ground_594/1 -> Subsystem9/18(Md18HoldReq)
  Ground_595/1 -> Subsystem9/19(Md19HoldReq)
  Ground_596/1 -> Subsystem9/20(Md20HoldReq)
  Ground_597/1 -> Subsystem9/21(Md21HoldReq)
  Ground_598/1 -> Subsystem9/22(Md22HoldReq)
  Ground_599/1 -> Subsystem9/23(Md23HoldReq)
  Ground_600/1 -> Subsystem9/24(Md24HoldReq)
  [Md56Stop] -> Subsystem9/25(Md25HoldReq)
  Ground_602/1 -> Subsystem9/26(Md26HoldReq)
  Ground_605/1 -> Subsystem9/29(Md29HoldReq)
  Ground_606/1 -> Subsystem9/30(Md30HoldReq)
  Ground_607/1 -> Subsystem9/31(Md31HoldReq)
  [R3LMdSeatOccupied] -> Subsystem9/32(Md32HoldReq)
  R2RMdSeatOccupied_Val_read/1 -> [R2RMdSeatOccupied]
  R2LMdSeatOccupied_Val_read/1 -> [R2LMdSeatOccupied]
  Logical Operator10/1 -> Subsystem18/28(Md28HoldReq)
  Subsystem19/1(ChldLkRspFlgR_Val_write) -> [ChldLkRspFlgR3L]
  [ChldLkRspFlgR3L] -> Logical Operator2/1
  [R3LMdSeatOccupied] -> Logical Operator2/2
  [ChldLkRspFlgR3L] -> Logical Operator5/1
  [R3LMdSeatOccupied] -> Logical Operator5/2
  [ChldLkRspFlgL] -> Logical Operator2/3
  Ground_30/1 -> Subsystem17/2(Md2HoldReq)
  [PassSeatOccupied] -> Logical Operator8/1
  Logical Operator8/1 -> Subsystem/28(Md28HoldReq)
  Logical Operator11/1 -> Subsystem1/28(Md28HoldReq)
  [ChldLkRspFlgR] -> Logical Operator13/1
  StNumFlg_Is7s_read/1 -> [is7s]
  [Md12Stop] -> Subsystem14/12(Md12HoldReq)
  Ground_12/1 -> Subsystem11/32(Md32HoldReq)
  IfVeSMSbThdRwLtStCshnFldUpwdDnwdMovConfig_Val_read/1 -> [ThdRwLtStCshnFldUpwdDnwdMovConfig]
  IfVeSMSuThdRwLtStCshnFldUpwdDnwdPos_Val_read/1 -> [ThdRwLtStCshnFldUpwdDnwdPos]
  IfVeSMSuThdRwRtStCshnFldUpwdDnwdPos_Val_read/1 -> [ThdRwRtStCshnFldUpwdDnwdPos]
  IfVeSMSbThdRwRtStCshnFldUpwdDnwdMovConfig_Val_read/1 -> [ThdRwRtStCshnFldUpwdDnwdMovConfig]
  [R3LMdSeatOccupied] -> Logical Operator84/2
  [ThdRwLtStCshnFldUpwdDnwdMovConfig] -> Logical Operator85/2
  Constant3/1 -> Relational Operator3/2
  [ThdRwLtStCshnFldUpwdDnwdPos] -> Relational Operator3/1
  Logical Operator85/1 -> Logical Operator84/3
  Relational Operator3/1 -> Logical Operator85/3
  [ChldLkRspFlgR3L] -> Logical Operator84/1
  Logical Operator86/1 -> Logical Operator85/1
  Logical Operator84/1 -> [Md8Stop]
  [ThdRwRtStCshnFldUpwdDnwdPos] -> Relational Operator1/1
  [Md8Stop] -> Subsystem3/8(Md8HoldReq)
  IfVeSMSuSecRwLtStBkReclnUpwdDnwdPos_Val_read/1 -> [IfVeSMSuSecRwLtStBkReclnUpwdDnwdPos]
  IfVeSMSuSecRwRtStBkReclnUpwdDnwdPos_Val_read/1 -> [IfVeSMSuSecRwRtStBkReclnUpwdDnwdPos]
  Md8R2LBkReclnUpwdDnwdTrgtPosCalib_TrgtPosArray_read/1 -> Demux/1
  Demux/1 -> [Md8R2LBkReclnUpwdDnwdTrgtPos]
  Md8R2RBkReclnUpwdDnwdTrgtPosCalib_TrgtPosArray_read/1 -> Demux1/1
  Demux1/1 -> [Md8R2RBkReclnUpwdDnwdTrgtPos]
  Md9R2RBkReclnUpwdDnwdTrgtPosCalib_TrgtPosArray_read/1 -> Demux2/1
  Demux2/1 -> [Md9R2RBkReclnUpwdDnwdTrgtPos]
  Demux1/2 -> Terminator/1
  Demux1/3 -> Terminator1/1
  Demux2/2 -> Terminator2/1
  Demux2/3 -> Terminator3/1
  Demux/2 -> Terminator4/1
  Demux/3 -> Terminator5/1
  [IfVeSMSuSecRwLtStBkReclnUpwdDnwdPos] -> Relational Operator4/1
  [Md8R2LBkReclnUpwdDnwdTrgtPos] -> Relational Operator4/2
  Relational Operator4/1 -> Logical Operator6/2
  Relational Operator5/1 -> Logical Operator7/2
  [IfVeSMSuSecRwRtStBkReclnUpwdDnwdPos] -> Relational Operator5/1
  [Md8R2RBkReclnUpwdDnwdTrgtPos] -> Relational Operator5/2
  [Md8Stop] -> Subsystem17/8(Md8HoldReq)
  [Md8Stop] -> Subsystem2/8(Md8HoldReq)
  [Md8Stop] -> Subsystem16/8(Md8HoldReq)
  [Md8Stop] -> Subsystem9/8(Md8HoldReq)
  [Md8Stop] -> Subsystem12/8(Md8HoldReq)
  [R3LMdSeatOccupied] -> Logical Operator3/3
  [R2RMdSeatOccupied] -> Logical Operator3/1
  [R2LMdSeatOccupied] -> Logical Operator3/2
  [R3RMdSeatOccupied] -> Logical Operator3/4
  [ChldLkRspFlgL] -> Subsystem17/1(Md1HoldReq)
  [ThdRwRtStCshnFldUpwdDnwdMovConfig] -> Logical Operator78/2
  Relational Operator1/1 -> Logical Operator78/3
  Constant1/1 -> Relational Operator1/2
  [Md9R2RBkReclnUpwdDnwdTrgtPos] -> Relational Operator2/2
  [IfVeSMSuSecRwRtStBkReclnUpwdDnwdPos] -> Relational Operator2/1
  Relational Operator2/1 -> Logical Operator78/4
  [ChldLkRspFlgR] -> Logical Operator78/1
  Logical Operator78/1 -> Logical Operator79/2
  [R3RMdSeatOccupied] -> Logical Operator79/1
  [Md9Stop] -> Subsystem4/9(Md9HoldReq)
  [Md9Stop] -> Subsystem11/9(Md9HoldReq)
  [Md9Stop] -> Subsystem10/9(Md9HoldReq)
  Logical Operator83/1 -> Logical Operator81/2
  [is7s] -> Logical Operator83/2
  Logical Operator81/1 -> [Md12Stop]
  [is7s] -> Switch19/2
  [ChldLkRspFlgR] -> Logical Operator81/1
  Switch19/1 -> Logical Operator81/3
  [R3LMdSeatOccupied] -> Logical Operator82/1
  Logical Operator82/1 -> Switch19/1
  [ChldLkRspFlgR3L] -> Logical Operator83/1
  [R3RMdSeatOccupied] -> Switch19/3
  [R3RMdSeatOccupied] -> Logical Operator82/2
  [Md12Stop] -> Subsystem1/12(Md12HoldReq)
  [Md12Stop] -> Subsystem/12(Md12HoldReq)
  [Md12Stop] -> Subsystem17/12(Md12HoldReq)
  [Md12Stop] -> Subsystem16/12(Md12HoldReq)
  [Md12Stop] -> Subsystem3/12(Md12HoldReq)
  [Md12Stop] -> Subsystem15/12(Md12HoldReq)
  [Md12Stop] -> Subsystem4/12(Md12HoldReq)
  [Md12Stop] -> Subsystem5/12(Md12HoldReq)
  [Md12Stop] -> Subsystem13/12(Md12HoldReq)
  [Md12Stop] -> Subsystem9/12(Md12HoldReq)
  [Md12Stop] -> Subsystem7/12(Md12HoldReq)
  [Md12Stop] -> Subsystem12/12(Md12HoldReq)
  [Md12Stop] -> Subsystem8/12(Md12HoldReq)
  [Md12Stop] -> Subsystem11/12(Md12HoldReq)
  [Md12Stop] -> Subsystem10/12(Md12HoldReq)
  ThdRwLtStChldLkReq_Val_read/1 -> Subsystem19/1(IfVeSMSeSecRwRtStChldLkRsp_Val_read)
  [PassSeatOccupied] -> Logical Operator10/1
  [is7s] -> Logical Operator45/2
  [ChldLkRspFlgR3L] -> Logical Operator45/1
  Logical Operator45/1 -> Logical Operator13/2
  [ChldLkRspFlgL] -> Logical Operator46/1
  [ChldLkRspFlgR3L] -> Logical Operator46/2
  Logical Operator46/1 -> [Md27Stop]
  [Md27Stop] -> Subsystem2/27(Md27HoldReq)
  [Md27Stop] -> Subsystem/27(Md27HoldReq)
  Logical Operator13/1 -> [Md28Stop]
  [Md28Stop] -> Subsystem2/28(Md28HoldReq)
  [Md28Stop] -> Subsystem16/28(Md28HoldReq)
  [Md28Stop] -> Subsystem17/28(Md28HoldReq)
  [Md28Stop] -> Subsystem3/28(Md28HoldReq)
  [Md27Stop] -> Subsystem3/27(Md27HoldReq)
  [Md27Stop] -> Subsystem15/27(Md27HoldReq)
  [Md28Stop] -> Subsystem15/28(Md28HoldReq)
  [Md27Stop] -> Subsystem4/27(Md27HoldReq)
  [Md28Stop] -> Subsystem4/28(Md28HoldReq)
  [Md27Stop] -> Subsystem14/27(Md27HoldReq)
  [Md28Stop] -> Subsystem14/28(Md28HoldReq)
  [Md27Stop] -> Subsystem5/27(Md27HoldReq)
  [Md28Stop] -> Subsystem5/28(Md28HoldReq)
  [Md27Stop] -> Subsystem13/27(Md27HoldReq)
  [Md28Stop] -> Subsystem13/28(Md28HoldReq)
  [Md27Stop] -> Subsystem6/27(Md27HoldReq)
  [Md28Stop] -> Subsystem6/28(Md28HoldReq)
  [Md27Stop] -> Subsystem9/27(Md27HoldReq)
  [Md28Stop] -> Subsystem9/28(Md28HoldReq)
  [Md27Stop] -> Subsystem7/27(Md27HoldReq)
  [Md28Stop] -> Subsystem7/28(Md28HoldReq)
  [Md27Stop] -> Subsystem12/27(Md27HoldReq)
  [Md28Stop] -> Subsystem12/28(Md28HoldReq)
  [Md27Stop] -> Subsystem8/27(Md27HoldReq)
  [Md28Stop] -> Subsystem8/28(Md28HoldReq)
  [Md27Stop] -> Subsystem11/27(Md27HoldReq)
  [Md28Stop] -> Subsystem11/28(Md28HoldReq)
  [Md27Stop] -> Subsystem10/27(Md27HoldReq)
  [Md28Stop] -> Subsystem10/28(Md28HoldReq)
  [Md28Stop] -> Logical Operator10/2
  [Md28Stop] -> Logical Operator8/2
  [PassSeatOccupied] -> Logical Operator11/1
  [Md28Stop] -> Logical Operator11/2
  Subsystem20/1(MdXXHolder) -> MdXXHolderInfo_Val_write/1
  [Md12Stop] -> Subsystem20/12(Md12HoldReq)
  [Md1Stop] -> Subsystem20/1(Md1HoldReq)
  [Md8Stop] -> Subsystem20/8(Md8HoldReq)
  [Md9Stop] -> Subsystem20/9(Md9HoldReq)
  [Md28Stop] -> Subsystem20/28(Md28HoldReq)
  [Md27Stop] -> Subsystem20/27(Md27HoldReq)
  Logical Operator2/1 -> [Md10Stop]
  [Md10Stop] -> Subsystem17/10(Md10HoldReq)
  [Md10Stop] -> Subsystem2/10(Md10HoldReq)
  [Md10Stop] -> Subsystem15/10(Md10HoldReq)
  [Md10Stop] -> Subsystem5/10(Md10HoldReq)
  [Md10Stop] -> Subsystem6/10(Md10HoldReq)
  [Md10Stop] -> Subsystem1/10(Md10HoldReq)
  [Md10Stop] -> Subsystem20/10(Md10HoldReq)
  Ground/1 -> Subsystem20/2(Md2HoldReq)
  Ground1/1 -> Subsystem20/3(Md3HoldReq)
  Ground2/1 -> Subsystem20/4(Md4HoldReq)
  Ground3/1 -> Subsystem20/5(Md5HoldReq)
  [Md61Stop] -> Subsystem20/6(Md6HoldReq)
  [Md11Stop] -> Subsystem20/11(Md11HoldReq)
  [Md13Stop] -> Subsystem20/13(Md13HoldReq)
  Ground8/1 -> Subsystem20/14(Md14HoldReq)
  Ground9/1 -> Subsystem20/15(Md15HoldReq)
  Ground10/1 -> Subsystem20/16(Md16HoldReq)
  Ground11/1 -> Subsystem20/17(Md17HoldReq)
  [Md53Stop] -> Subsystem20/18(Md18HoldReq)
  Ground13/1 -> Subsystem20/19(Md19HoldReq)
  Ground14/1 -> Subsystem20/20(Md20HoldReq)
  Ground15/1 -> Subsystem20/21(Md21HoldReq)
  Ground16/1 -> Subsystem20/22(Md22HoldReq)
  Ground17/1 -> Subsystem20/23(Md23HoldReq)
  Ground18/1 -> Subsystem20/24(Md24HoldReq)
  [Md56Stop] -> Subsystem20/25(Md25HoldReq)
  Ground20/1 -> Subsystem20/26(Md26HoldReq)
  Ground21/1 -> Subsystem20/29(Md29HoldReq)
  [PassSeatOccupied] -> Subsystem20/30(Md30HoldReq)
  Ground23/1 -> Subsystem20/31(Md31HoldReq)
  [Md32Stop] -> Subsystem20/32(Md32HoldReq)
  Constant/1 -> [Md1Stop]
  [R3RMdSeatOccupied] -> Logical Operator1/2
  [R3LMdSeatOccupied] -> Logical Operator1/1
  Logical Operator1/1 -> [Md56Stop]
  Logical Operator3/1 -> Terminator6/1
  [ChldLkRspFlgL] -> Logical Operator6/1
  Logical Operator6/1 -> Logical Operator86/1
  Logical Operator7/1 -> Logical Operator86/2
  [ChldLkRspFlgR] -> Logical Operator7/1
  [ChldLkRspFlgL] -> [Md11Stop]
  [ChldLkRspFlgR] -> [Md13Stop]
  [ChldLkRspFlgR3L] -> Logical Operator9/1
  Logical Operator9/1 -> [Md32Stop]
  [ChldLkRspFlgL] -> Logical Operator12/1
  Logical Operator12/1 -> Logical Operator9/2
  [Md32R2LBkReclnUpwdDnwdTrgtPos1] -> Relational Operator6/2
  Relational Operator6/1 -> Logical Operator12/2
  [IfVeSMSuSecRwLtStBkReclnUpwdDnwdPos] -> Relational Operator6/1
  [IfVeSMSuSecRwRtStBkReclnUpwdDnwdPos] -> Relational Operator8/1
  Relational Operator8/1 -> Logical Operator14/2
  [Md53R2RBkReclnUpwdDnwdTrgtPos1] -> Relational Operator8/2
  [ChldLkRspFlgR] -> Logical Operator14/1
  KeSMSwAcsMd53SecRwRtStBkReclnUpwdDnwdPos1/1 -> [Md53R2RBkReclnUpwdDnwdTrgtPos1]
  KeSMSwAcsMd32SecRwLtStBkReclnUpwdDnwdPos1/1 -> [Md32R2LBkReclnUpwdDnwdTrgtPos1]
  [ChldLkRspFlgR] -> Logical Operator15/1
  [Md53R2RBkReclnUpwdDnwdTrgtPos1] -> Relational Operator7/2
  Relational Operator7/1 -> Logical Operator15/2
  [IfVeSMSuSecRwRtStBkReclnUpwdDnwdPos] -> Relational Operator7/1
  Logical Operator15/1 -> Logical Operator9/3
  [R3LMdSeatOccupied] -> Logical Operator9/4
  Logical Operator14/1 -> Logical Operator16/1
  Logical Operator16/1 -> [Md53Stop]
  [R3RMdSeatOccupied] -> Logical Operator16/2
  Logical Operator/1 -> Subsystem17/25(Md25HoldReq)
  [Md56Stop] -> Logical Operator/2
  [ChldLkRspFlgL] -> Logical Operator/1
  Logical Operator17/1 -> Subsystem4/25(Md25HoldReq)
  [Md56Stop] -> Logical Operator17/2
  [ChldLkRspFlgR] -> Logical Operator17/1
  [ChldLkRspFlgR] -> Subsystem4/1(Md1HoldReq)
  [ChldLkRspFlgL] -> Logical Operator4/1
  [ChldLkRspFlgR] -> Logical Operator4/2
  [ChldLkRspFlgR3L] -> Logical Operator4/3
  Logical Operator4/1 -> [Md61Stop]
  Logical Operator18/1 -> Logical Operator4/4
  Logical Operator21/1 -> Logical Operator4/5
  Logical Operator22/1 -> Logical Operator4/6
  Md61PassStTrgtIsFld_Val_read/1 -> Logical Operator18/1
  [PassSeatOccupied] -> Logical Operator18/2
  Logical Operator24/1 -> Logical Operator19/6
  Logical Operator23/1 -> Logical Operator19/5
  Logical Operator20/1 -> Logical Operator19/4
  Logical Operator19/1 -> [Md62Stop]
  [ChldLkRspFlgR3L] -> Logical Operator19/3
  [ChldLkRspFlgR] -> Logical Operator19/2
  [ChldLkRspFlgL] -> Logical Operator19/1
  [PassSeatOccupied] -> Logical Operator20/2
  Md62PassStTrgtIsFld_Val_read/1 -> Logical Operator20/1
  Md61ThdRwLtStTrgtIsFld_Val_read/1 -> Logical Operator21/1
  Md61ThdRwRtStTrgtIsFld_Val_read/1 -> Logical Operator22/1
  [R3RMdSeatOccupied] -> Logical Operator22/2
  [R3LMdSeatOccupied] -> Logical Operator21/2
  [R3LMdSeatOccupied] -> Logical Operator23/2
  Md62ThdRwLtStTrgtIsFld_Val_read/1 -> Logical Operator23/1
  [R3RMdSeatOccupied] -> Logical Operator24/2
  Md62ThdRwRtStTrgtIsFld_Val_read/1 -> Logical Operator24/1
  [Md62Stop] -> Subsystem20/7(Md7HoldReq)
  Unit Delay/1 -> Compare To Constant/1
  BkReclinctrlquitflagL_Val_read/1 -> Unit Delay/1, Compare To Constant1/1
  Compare To Constant/1 -> Logical Operator25/1
  Compare To Constant1/1 -> Logical Operator25/2
  Logical Operator25/1 -> Logical Operator2/4
  Unit Delay1/1 -> Compare To Constant2/1
  FwdBkwdquitflagL_Val_read/1 -> Compare To Constant3/1, Unit Delay1/1
  Compare To Constant3/1 -> Logical Operator26/2
  Compare To Constant2/1 -> Logical Operator26/1
  Logical Operator26/1 -> Logical Operator2/5
  Unit Delay2/1 -> Compare To Constant4/1
  LgrstDwwdUpwdquitflagL_Val_read/1 -> Unit Delay2/1, Compare To Constant5/1
  Compare To Constant5/1 -> Logical Operator27/2
  Compare To Constant4/1 -> Logical Operator27/1
  Logical Operator27/1 -> Logical Operator2/6
  Unit Delay3/1 -> Compare To Constant6/1
  LgrstInwdOtwdquitflagL_Val_read/1 -> Unit Delay3/1, Compare To Constant7/1
  Compare To Constant7/1 -> Logical Operator28/2
  Compare To Constant6/1 -> Logical Operator28/1
  Logical Operator28/1 -> Logical Operator2/8
  Unit Delay4/1 -> Compare To Constant8/1
  zeroquitflagL_Val_read/1 -> Unit Delay4/1, Compare To Constant9/1
  Compare To Constant9/1 -> Logical Operator29/2
  Compare To Constant8/1 -> Logical Operator29/1
  Logical Operator29/1 -> Logical Operator2/7
  Unit Delay5/1 -> Compare To Constant10/1
  BkReclnquitflag_Val_read/1 -> Unit Delay5/1, Compare To Constant11/1
  Compare To Constant11/1 -> Logical Operator30/2
  Compare To Constant10/1 -> Logical Operator30/1
  Logical Operator30/1 -> Logical Operator81/4
  Unit Delay6/1 -> Compare To Constant12/1
  LgrstInwrdOutwdquitflag_Val_read/1 -> Unit Delay6/1, Compare To Constant13/1
  Compare To Constant13/1 -> Logical Operator31/2
  Compare To Constant12/1 -> Logical Operator31/1
  Logical Operator31/1 -> Logical Operator81/6
  Unit Delay7/1 -> Compare To Constant14/1
  FwdBkwdquitflag_Val_read/1 -> Unit Delay7/1, Compare To Constant15/1
  Compare To Constant15/1 -> Logical Operator32/2
  Compare To Constant14/1 -> Logical Operator32/1
  Logical Operator32/1 -> Logical Operator81/5
  Unit Delay8/1 -> Compare To Constant16/1
  Zeroquitflag_Val_read/1 -> Unit Delay8/1, Compare To Constant17/1
  Compare To Constant17/1 -> Logical Operator33/2
  Compare To Constant16/1 -> Logical Operator33/1
  Logical Operator33/1 -> Logical Operator81/7
  Unit Delay9/1 -> Compare To Constant18/1
  LgrstUpwdDnwdquitflag_Val_read/1 -> Unit Delay9/1, Compare To Constant19/1
  Compare To Constant19/1 -> Logical Operator34/2
  Compare To Constant18/1 -> Logical Operator34/1
  Logical Operator34/1 -> Logical Operator81/8
  modestate32_Val_read/1 -> Subsystem20/33(modestate32_Val_read)
